simulink model "entire_leg_assembly"  (R2023b)
settings: Solver=ode15s  StartTime=0.0  StopTime=3*(2*length(Wp_1_forward_U)/10)  FixedStep=0.1  MaxStep=1e-3  RelTol=1e-2  AbsTol=1e-5  EnableMultiTasking=on
values from neighbouring files (symbols this model uses):
  Theta1_initial_value = wp_swing(1,1)    [Input_joint_angles.m]
  Theta2_initial_value = wp_swing(2,1)    [Input_joint_angles.m]
  Wp_1_forward_L_3 = repmat(Wp_1_forward_L, 1, 10)    [Input_joint_angles.m]
  Wp_1_forward_U_3 = repmat(Wp_1_forward_U, 1, 10)    [Input_joint_angles.m]
  Wp_3_backward_L_3 = repmat(Wp_3_forward_L, 1, 10)    [Input_joint_angles.m]
  Wp_3_backward_U_3 = repmat(Wp_3_forward_U, 1, 10)    [Input_joint_angles.m]
  Wp_3_forward_L_3 = [1.04719759763 1.04719759763 1.04719759763 1.04719759763 1.04719759763 1.04719759763 1.31601388737 1.31601388737 1.04719759763 1.04719759763 1.04719759763 1.31601388737 ... (1800 elements, 6x300)]    [ForwardWalk.mat]
  Wp_3_forward_U_3 = [-0.523598776024 -0.523598776024 -0.523598776024 -0.523598776024 -0.523598776024 -0.523598776024 -0.649667510569 -0.649667510569 -0.523598776024 -0.523598776024 -0.523598776024 -0.649667510569 ... (1800 elements, 6x300)]    [ForwardWalk.mat]
undefined symbols (not defined in the file or in its folder): X, Y, Z
libraries: sm_lib x76, nesl_utility x25
(part 3 of 3)

== system entire_leg_assembly/Leg3/Leg_LR/Lower_limb1 ==
  Lower_limb : sm_lib/Body Elements/File Solid  Commented=on  ExtGeomFileName=C:\summer 23 thesis om\Robot assembly with 2 linear actuators\Simscape_demo\Leg_lower.STL  UnitType=Custom  ExtGeomFileUnits=mm  StepReaderType=HEX  ExportConvexHullGeometry=off  InertiaType=CalculateFromGeometry  Mass=1.6  MassUnits=kg  CenterOfMass=[0 0 0]  CenterOfMassUnits=m  MomentsOfInertia=[1 1 1]  MomentsOfInertiaUnits=kg*m^2  ProductsOfInertia=[0 0 0]  ProductsOfInertiaUnits=kg*m^2  BasedOnType=Mass  Density=1000  DensityUnits=kg/m^3  DoExposeReferenceFrame=on  SerializedFrames=<Frames><Frame><Id>Frame1</Id><Value><Name>F1</Name><Origin><Source>CenterOfMassFrame</Source><FeatureName></FeatureName></Origin><PrimaryAxis><DefinedDirection>-Y</DefinedDirection><Source>ReferenceFrame</Source><SourceDirection>+Z</SourceDirection><FeatureName></FeatureName></PrimaryAxis><SecondaryAxis><DefinedDirection>+X</DefinedDirection><Source>ReferenceFrame</Source><SourceDirection>+X</SourceDirection><FeatureName></FeatureName></SecondaryAxis></Value></Frame></Frames>  GraphicType=FromGeometry  MarkerShape=Sphere  MarkerSize=10  GraphicVisPropType=SimpleVisualProperties  GraphicDiffuseColor=[0.5 0.5 0.5]  GraphicSpecularColor=[0.5 0.5 0.5 1.0]  GraphicAmbientColor=[0.15 0.15 0.15 1.0]  GraphicEmissiveColor=[0.0 0.0 0.0 1.0]  GraphicShininess=75  GraphicOpacity=1.0
  Lower_limb_OLD : sm_lib/Body Elements/Cylindrical Solid  GraphicAmbientColor=[0.15 0.15 0.15 1.0]  BasedOnType=Density  CenterOfMass=[0 0 0]  CenterOfMassUnits=m  GraphicDiffuseColor=[0.5 0.5 0.5]  CylinderLength=6  CylinderLengthUnits=ft  CylinderRadius=17.46  CylinderRadiusUnits=mm  Density=3000  DensityUnits=kg/m^3  DoExposeReferenceFrame=on  GraphicEmissiveColor=[0.0 0.0 0.0 1.0]  ExportEntireGeometry=on  SerializedFrames=<Frames><Frame><Id>Frame1</Id><Value><Name>F1</Name><Origin><Source>ReferenceFrame</Source><FeatureName></FeatureName></Origin><PrimaryAxis><DefinedDirection>+Y</DefinedDirection><Source>ReferenceFrame</Source><SourceDirection>+Z</SourceDirection><FeatureName></FeatureName></PrimaryAxis><SecondaryAxis><DefinedDirection>+X</DefinedDirection><Source>ReferenceFrame</Source><SourceDirection>+X</SourceDirection><FeatureName></FeatureName></SecondaryAxis></Value></Frame></Frames>  MarkerShape=Sphere  MarkerSize=10  GraphicType=FromGeometry  InertiaType=CalculateFromGeometry  Mass=1  MassUnits=kg  MomentsOfInertia=[1 1 1]  MomentsOfInertiaUnits=kg*m^2  GraphicOpacity=1.0  ProductsOfInertia=[0 0 0]  ProductsOfInertiaUnits=kg*m^2  GraphicShininess=75  GraphicSpecularColor=[0.5 0.5 0.5 1.0]  GraphicVisPropType=SimpleVisualProperties
  Rigid Transform2 : sm_lib/Frames and Transforms/Rigid Transform  TranslationMethod=Cartesian  TranslationStandardOffset=0  TranslationStandardOffsetUnits=m  TranslationStandardAxis=+Z  TranslationCartesianOffset=[0 -3 0]  TranslationCartesianOffsetUnits=ft  TranslationROffset=0  TranslationROffsetUnits=m  TranslationZOffset=0  TranslationZOffsetUnits=m  TranslationThetaOffset=0  TranslationThetaOffsetUnits=deg  RotationMethod=None  RotationAngleUnits=deg  RotationStandardAxis=+Y  RotationAngle=0  RotationArbitraryAxis=[0 0 1]  FollAlignAxisA=+X  BaseAlignAxisA=+Y  FollAlignAxisB=+Y  BaseAlignAxisB=+Z  RotationSequenceAxes=FollowerAxes  RotationSequence=XYX  RotationSequenceAngles=[0 0 0]  RotationSequenceAnglesUnits=deg  RotationMatrix=[1 0 0; 0 1 0; 0 0 1]  Quaternion=[1 0 0 0]
  Conn1 : PMIOPort  Side=Left
  Conn2 : PMIOPort  Port=2  Side=Left
  connections:
  Conn1/RConn1 -- Rigid Transform2/LConn1
  Rigid Transform2/RConn1 -- Lower_limb_OLD/LConn1
  Conn2/RConn1 -- Lower_limb_OLD/LConn2

== system entire_leg_assembly/Leg3/Leg_LR/Upper_limb1 ==
  Rigid Transform : sm_lib/Frames and Transforms/Rigid Transform  TranslationMethod=Cartesian  TranslationStandardOffset=0  TranslationStandardOffsetUnits=m  TranslationStandardAxis=+Z  TranslationCartesianOffset=[0 -3 0]  TranslationCartesianOffsetUnits=ft  TranslationROffset=0  TranslationROffsetUnits=m  TranslationZOffset=0  TranslationZOffsetUnits=m  TranslationThetaOffset=0  TranslationThetaOffsetUnits=deg  RotationMethod=None  RotationAngleUnits=deg  RotationStandardAxis=+Y  RotationAngle=90  RotationArbitraryAxis=[0 0 1]  FollAlignAxisA=+X  BaseAlignAxisA=+Y  FollAlignAxisB=+Y  BaseAlignAxisB=+Z  RotationSequenceAxes=FollowerAxes  RotationSequence=XYX  RotationSequenceAngles=[0 0 0]  RotationSequenceAnglesUnits=deg  RotationMatrix=[1 0 0; 0 1 0; 0 0 1]  Quaternion=[1 0 0 0]
  Rigid Transform1 : sm_lib/Frames and Transforms/Rigid Transform  TranslationMethod=Cartesian  TranslationStandardOffset=0  TranslationStandardOffsetUnits=m  TranslationStandardAxis=+Z  TranslationCartesianOffset=[0 -3 0]  TranslationCartesianOffsetUnits=ft  TranslationROffset=0  TranslationROffsetUnits=m  TranslationZOffset=0  TranslationZOffsetUnits=m  TranslationThetaOffset=0  TranslationThetaOffsetUnits=deg  RotationMethod=None  RotationAngleUnits=deg  RotationStandardAxis=+Z  RotationAngle=0.0  RotationArbitraryAxis=[0 0 1]  FollAlignAxisA=+X  BaseAlignAxisA=+Y  FollAlignAxisB=+Y  BaseAlignAxisB=+Z  RotationSequenceAxes=FollowerAxes  RotationSequence=XYX  RotationSequenceAngles=[0 0 0]  RotationSequenceAnglesUnits=deg  RotationMatrix=[1 0 0; 0 1 0; 0 0 1]  Quaternion=[1 0 0 0]
  Upper_limb : sm_lib/Body Elements/File Solid  ExtGeomFileName=C:\summer 23 thesis om\Robot assembly with 2 linear actuators\Simscape_demo\Leg_upper.STL  UnitType=Custom  ExtGeomFileUnits=mm  StepReaderType=HEX  ExportConvexHullGeometry=off  InertiaType=CalculateFromGeometry  Mass=1.6  MassUnits=kg  CenterOfMass=[0 0 0]  CenterOfMassUnits=m  MomentsOfInertia=[1 1 1]  MomentsOfInertiaUnits=kg*m^2  ProductsOfInertia=[0 0 0]  ProductsOfInertiaUnits=kg*m^2  BasedOnType=Mass  Density=1000  DensityUnits=kg/m^3  DoExposeReferenceFrame=on  SerializedFrames=<Frames><Frame><Id>Frame1</Id><Value><Name>F1</Name><Origin><Source>CenterOfMassFrame</Source><FeatureName></FeatureName></Origin><PrimaryAxis><DefinedDirection>-Y</DefinedDirection><Source>ReferenceFrame</Source><SourceDirection>+Z</SourceDirection><FeatureName></FeatureName></PrimaryAxis><SecondaryAxis><DefinedDirection>+X</DefinedDirection><Source>ReferenceFrame</Source><SourceDirection>+X</SourceDirection><FeatureName></FeatureName></SecondaryAxis></Value></Frame></Frames>  GraphicType=FromGeometry  MarkerShape=Sphere  MarkerSize=10  GraphicVisPropType=SimpleVisualProperties  GraphicDiffuseColor=[0.5 0.5 0.5]  GraphicSpecularColor=[0.5 0.5 0.5 1.0]  GraphicAmbientColor=[0.15 0.15 0.15 1.0]  GraphicEmissiveColor=[0.0 0.0 0.0 1.0]  GraphicShininess=75  GraphicOpacity=1.0
  Conn1 : PMIOPort  Side=Left
  Conn2 : PMIOPort  Port=2  Side=Right
  connections:
  Rigid Transform/LConn1 -- Conn1/RConn1
  Conn2/RConn1 -- Rigid Transform1/RConn1
  Rigid Transform1/LConn1 -- Upper_limb/LConn1 -- Rigid Transform/RConn1

== system entire_leg_assembly/Leg4/Leg_RF/Lower_limb1 ==
  Lower_limb : sm_lib/Body Elements/File Solid  Commented=on  ExtGeomFileName=C:\summer 23 thesis om\Robot assembly with 2 linear actuators\Simscape_demo\Leg_lower.STL  UnitType=Custom  ExtGeomFileUnits=mm  StepReaderType=HEX  ExportConvexHullGeometry=off  InertiaType=CalculateFromGeometry  Mass=1.6  MassUnits=kg  CenterOfMass=[0 0 0]  CenterOfMassUnits=m  MomentsOfInertia=[1 1 1]  MomentsOfInertiaUnits=kg*m^2  ProductsOfInertia=[0 0 0]  ProductsOfInertiaUnits=kg*m^2  BasedOnType=Mass  Density=1000  DensityUnits=kg/m^3  DoExposeReferenceFrame=on  SerializedFrames=<Frames><Frame><Id>Frame1</Id><Value><Name>F1</Name><Origin><Source>CenterOfMassFrame</Source><FeatureName></FeatureName></Origin><PrimaryAxis><DefinedDirection>-Y</DefinedDirection><Source>ReferenceFrame</Source><SourceDirection>+Z</SourceDirection><FeatureName></FeatureName></PrimaryAxis><SecondaryAxis><DefinedDirection>+X</DefinedDirection><Source>ReferenceFrame</Source><SourceDirection>+X</SourceDirection><FeatureName></FeatureName></SecondaryAxis></Value></Frame></Frames>  GraphicType=FromGeometry  MarkerShape=Sphere  MarkerSize=10  GraphicVisPropType=SimpleVisualProperties  GraphicDiffuseColor=[0.5 0.5 0.5]  GraphicSpecularColor=[0.5 0.5 0.5 1.0]  GraphicAmbientColor=[0.15 0.15 0.15 1.0]  GraphicEmissiveColor=[0.0 0.0 0.0 1.0]  GraphicShininess=75  GraphicOpacity=1.0
  Lower_limb_OLD : sm_lib/Body Elements/Cylindrical Solid  GraphicAmbientColor=[0.15 0.15 0.15 1.0]  BasedOnType=Density  CenterOfMass=[0 0 0]  CenterOfMassUnits=m  GraphicDiffuseColor=[0.5 0.5 0.5]  CylinderLength=6  CylinderLengthUnits=ft  CylinderRadius=17.46  CylinderRadiusUnits=mm  Density=3000  DensityUnits=kg/m^3  DoExposeReferenceFrame=on  GraphicEmissiveColor=[0.0 0.0 0.0 1.0]  ExportEntireGeometry=on  SerializedFrames=<Frames><Frame><Id>Frame1</Id><Value><Name>F1</Name><Origin><Source>ReferenceFrame</Source><FeatureName></FeatureName></Origin><PrimaryAxis><DefinedDirection>+Y</DefinedDirection><Source>ReferenceFrame</Source><SourceDirection>+Z</SourceDirection><FeatureName></FeatureName></PrimaryAxis><SecondaryAxis><DefinedDirection>+X</DefinedDirection><Source>ReferenceFrame</Source><SourceDirection>+X</SourceDirection><FeatureName></FeatureName></SecondaryAxis></Value></Frame></Frames>  MarkerShape=Sphere  MarkerSize=10  GraphicType=FromGeometry  InertiaType=CalculateFromGeometry  Mass=1  MassUnits=kg  MomentsOfInertia=[1 1 1]  MomentsOfInertiaUnits=kg*m^2  GraphicOpacity=1.0  ProductsOfInertia=[0 0 0]  ProductsOfInertiaUnits=kg*m^2  GraphicShininess=75  GraphicSpecularColor=[0.5 0.5 0.5 1.0]  GraphicVisPropType=SimpleVisualProperties
  Rigid Transform2 : sm_lib/Frames and Transforms/Rigid Transform  TranslationMethod=Cartesian  TranslationStandardOffset=0  TranslationStandardOffsetUnits=m  TranslationStandardAxis=+Z  TranslationCartesianOffset=[0 -3 0]  TranslationCartesianOffsetUnits=ft  TranslationROffset=0  TranslationROffsetUnits=m  TranslationZOffset=0  TranslationZOffsetUnits=m  TranslationThetaOffset=0  TranslationThetaOffsetUnits=deg  RotationMethod=None  RotationAngleUnits=deg  RotationStandardAxis=+Y  RotationAngle=0  RotationArbitraryAxis=[0 0 1]  FollAlignAxisA=+X  BaseAlignAxisA=+Y  FollAlignAxisB=+Y  BaseAlignAxisB=+Z  RotationSequenceAxes=FollowerAxes  RotationSequence=XYX  RotationSequenceAngles=[0 0 0]  RotationSequenceAnglesUnits=deg  RotationMatrix=[1 0 0; 0 1 0; 0 0 1]  Quaternion=[1 0 0 0]
  Conn1 : PMIOPort  Side=Left
  Connection Port : PMIOPort  Port=2  Side=Left
  connections:
  Conn1/RConn1 -- Rigid Transform2/LConn1
  Rigid Transform2/RConn1 -- Lower_limb_OLD/LConn1
  Lower_limb_OLD/LConn2 -- Connection Port/RConn1

== system entire_leg_assembly/Leg4/Leg_RF/Upper_limb1 ==
  Rigid Transform : sm_lib/Frames and Transforms/Rigid Transform  TranslationMethod=Cartesian  TranslationStandardOffset=0  TranslationStandardOffsetUnits=m  TranslationStandardAxis=+Z  TranslationCartesianOffset=[0 -3 0]  TranslationCartesianOffsetUnits=ft  TranslationROffset=0  TranslationROffsetUnits=m  TranslationZOffset=0  TranslationZOffsetUnits=m  TranslationThetaOffset=0  TranslationThetaOffsetUnits=deg  RotationMethod=None  RotationAngleUnits=deg  RotationStandardAxis=+Y  RotationAngle=90  RotationArbitraryAxis=[0 0 1]  FollAlignAxisA=+X  BaseAlignAxisA=+Y  FollAlignAxisB=+Y  BaseAlignAxisB=+Z  RotationSequenceAxes=FollowerAxes  RotationSequence=XYX  RotationSequenceAngles=[0 0 0]  RotationSequenceAnglesUnits=deg  RotationMatrix=[1 0 0; 0 1 0; 0 0 1]  Quaternion=[1 0 0 0]
  Rigid Transform1 : sm_lib/Frames and Transforms/Rigid Transform  TranslationMethod=Cartesian  TranslationStandardOffset=0  TranslationStandardOffsetUnits=m  TranslationStandardAxis=+Z  TranslationCartesianOffset=[0 -3 0]  TranslationCartesianOffsetUnits=ft  TranslationROffset=0  TranslationROffsetUnits=m  TranslationZOffset=0  TranslationZOffsetUnits=m  TranslationThetaOffset=0  TranslationThetaOffsetUnits=deg  RotationMethod=None  RotationAngleUnits=deg  RotationStandardAxis=+Z  RotationAngle=0.0  RotationArbitraryAxis=[0 0 1]  FollAlignAxisA=+X  BaseAlignAxisA=+Y  FollAlignAxisB=+Y  BaseAlignAxisB=+Z  RotationSequenceAxes=FollowerAxes  RotationSequence=XYX  RotationSequenceAngles=[0 0 0]  RotationSequenceAnglesUnits=deg  RotationMatrix=[1 0 0; 0 1 0; 0 0 1]  Quaternion=[1 0 0 0]
  Upper_limb : sm_lib/Body Elements/File Solid  ExtGeomFileName=C:\summer 23 thesis om\Robot assembly with 2 linear actuators\Simscape_demo\Leg_upper.STL  UnitType=Custom  ExtGeomFileUnits=mm  StepReaderType=HEX  ExportConvexHullGeometry=off  InertiaType=CalculateFromGeometry  Mass=1.6  MassUnits=kg  CenterOfMass=[0 0 0]  CenterOfMassUnits=m  MomentsOfInertia=[1 1 1]  MomentsOfInertiaUnits=kg*m^2  ProductsOfInertia=[0 0 0]  ProductsOfInertiaUnits=kg*m^2  BasedOnType=Mass  Density=1000  DensityUnits=kg/m^3  DoExposeReferenceFrame=on  SerializedFrames=<Frames><Frame><Id>Frame1</Id><Value><Name>F1</Name><Origin><Source>CenterOfMassFrame</Source><FeatureName></FeatureName></Origin><PrimaryAxis><DefinedDirection>-Y</DefinedDirection><Source>ReferenceFrame</Source><SourceDirection>+Z</SourceDirection><FeatureName></FeatureName></PrimaryAxis><SecondaryAxis><DefinedDirection>+X</DefinedDirection><Source>ReferenceFrame</Source><SourceDirection>+X</SourceDirection><FeatureName></FeatureName></SecondaryAxis></Value></Frame></Frames>  GraphicType=FromGeometry  MarkerShape=Sphere  MarkerSize=10  GraphicVisPropType=SimpleVisualProperties  GraphicDiffuseColor=[0.5 0.5 0.5]  GraphicSpecularColor=[0.5 0.5 0.5 1.0]  GraphicAmbientColor=[0.15 0.15 0.15 1.0]  GraphicEmissiveColor=[0.0 0.0 0.0 1.0]  GraphicShininess=75  GraphicOpacity=1.0
  Conn1 : PMIOPort  Side=Left
  Conn2 : PMIOPort  Port=2  Side=Right
  connections:
  Rigid Transform/LConn1 -- Conn1/RConn1
  Conn2/RConn1 -- Rigid Transform1/RConn1
  Rigid Transform1/LConn1 -- Upper_limb/LConn1 -- Rigid Transform/RConn1

== system entire_leg_assembly/Leg5/Leg_RM/Lower_limb1 ==
  Lower_limb : sm_lib/Body Elements/File Solid  Commented=on  ExtGeomFileName=C:\summer 23 thesis om\Robot assembly with 2 linear actuators\Simscape_demo\Leg_lower.STL  UnitType=Custom  ExtGeomFileUnits=mm  StepReaderType=HEX  ExportConvexHullGeometry=off  InertiaType=CalculateFromGeometry  Mass=1.6  MassUnits=kg  CenterOfMass=[0 0 0]  CenterOfMassUnits=m  MomentsOfInertia=[1 1 1]  MomentsOfInertiaUnits=kg*m^2  ProductsOfInertia=[0 0 0]  ProductsOfInertiaUnits=kg*m^2  BasedOnType=Mass  Density=1000  DensityUnits=kg/m^3  DoExposeReferenceFrame=on  SerializedFrames=<Frames><Frame><Id>Frame1</Id><Value><Name>F1</Name><Origin><Source>CenterOfMassFrame</Source><FeatureName></FeatureName></Origin><PrimaryAxis><DefinedDirection>-Y</DefinedDirection><Source>ReferenceFrame</Source><SourceDirection>+Z</SourceDirection><FeatureName></FeatureName></PrimaryAxis><SecondaryAxis><DefinedDirection>+X</DefinedDirection><Source>ReferenceFrame</Source><SourceDirection>+X</SourceDirection><FeatureName></FeatureName></SecondaryAxis></Value></Frame></Frames>  GraphicType=FromGeometry  MarkerShape=Sphere  MarkerSize=10  GraphicVisPropType=SimpleVisualProperties  GraphicDiffuseColor=[0.5 0.5 0.5]  GraphicSpecularColor=[0.5 0.5 0.5 1.0]  GraphicAmbientColor=[0.15 0.15 0.15 1.0]  GraphicEmissiveColor=[0.0 0.0 0.0 1.0]  GraphicShininess=75  GraphicOpacity=1.0
  Lower_limb_OLD : sm_lib/Body Elements/Cylindrical Solid  GraphicAmbientColor=[0.15 0.15 0.15 1.0]  BasedOnType=Density  CenterOfMass=[0 0 0]  CenterOfMassUnits=m  GraphicDiffuseColor=[0.5 0.5 0.5]  CylinderLength=6  CylinderLengthUnits=ft  CylinderRadius=17.46  CylinderRadiusUnits=mm  Density=3000  DensityUnits=kg/m^3  DoExposeReferenceFrame=on  GraphicEmissiveColor=[0.0 0.0 0.0 1.0]  ExportEntireGeometry=on  SerializedFrames=<Frames><Frame><Id>Frame1</Id><Value><Name>F1</Name><Origin><Source>ReferenceFrame</Source><FeatureName></FeatureName></Origin><PrimaryAxis><DefinedDirection>+Y</DefinedDirection><Source>ReferenceFrame</Source><SourceDirection>+Z</SourceDirection><FeatureName></FeatureName></PrimaryAxis><SecondaryAxis><DefinedDirection>+X</DefinedDirection><Source>ReferenceFrame</Source><SourceDirection>+X</SourceDirection><FeatureName></FeatureName></SecondaryAxis></Value></Frame></Frames>  MarkerShape=Sphere  MarkerSize=10  GraphicType=FromGeometry  InertiaType=CalculateFromGeometry  Mass=1  MassUnits=kg  MomentsOfInertia=[1 1 1]  MomentsOfInertiaUnits=kg*m^2  GraphicOpacity=1.0  ProductsOfInertia=[0 0 0]  ProductsOfInertiaUnits=kg*m^2  GraphicShininess=75  GraphicSpecularColor=[0.5 0.5 0.5 1.0]  GraphicVisPropType=SimpleVisualProperties
  Rigid Transform2 : sm_lib/Frames and Transforms/Rigid Transform  TranslationMethod=Cartesian  TranslationStandardOffset=0  TranslationStandardOffsetUnits=m  TranslationStandardAxis=+Z  TranslationCartesianOffset=[0 -3 0]  TranslationCartesianOffsetUnits=ft  TranslationROffset=0  TranslationROffsetUnits=m  TranslationZOffset=0  TranslationZOffsetUnits=m  TranslationThetaOffset=0  TranslationThetaOffsetUnits=deg  RotationMethod=None  RotationAngleUnits=deg  RotationStandardAxis=+Y  RotationAngle=0  RotationArbitraryAxis=[0 0 1]  FollAlignAxisA=+X  BaseAlignAxisA=+Y  FollAlignAxisB=+Y  BaseAlignAxisB=+Z  RotationSequenceAxes=FollowerAxes  RotationSequence=XYX  RotationSequenceAngles=[0 0 0]  RotationSequenceAnglesUnits=deg  RotationMatrix=[1 0 0; 0 1 0; 0 0 1]  Quaternion=[1 0 0 0]
  Conn1 : PMIOPort  Side=Left
  Connection Port : PMIOPort  Port=2  Side=Left
  connections:
  Conn1/RConn1 -- Rigid Transform2/LConn1
  Rigid Transform2/RConn1 -- Lower_limb_OLD/LConn1
  Lower_limb_OLD/LConn2 -- Connection Port/RConn1

== system entire_leg_assembly/Leg5/Leg_RM/Upper_limb1 ==
  Rigid Transform : sm_lib/Frames and Transforms/Rigid Transform  TranslationMethod=Cartesian  TranslationStandardOffset=0  TranslationStandardOffsetUnits=m  TranslationStandardAxis=+Z  TranslationCartesianOffset=[0 -3 0]  TranslationCartesianOffsetUnits=ft  TranslationROffset=0  TranslationROffsetUnits=m  TranslationZOffset=0  TranslationZOffsetUnits=m  TranslationThetaOffset=0  TranslationThetaOffsetUnits=deg  RotationMethod=None  RotationAngleUnits=deg  RotationStandardAxis=+Y  RotationAngle=90  RotationArbitraryAxis=[0 0 1]  FollAlignAxisA=+X  BaseAlignAxisA=+Y  FollAlignAxisB=+Y  BaseAlignAxisB=+Z  RotationSequenceAxes=FollowerAxes  RotationSequence=XYX  RotationSequenceAngles=[0 0 0]  RotationSequenceAnglesUnits=deg  RotationMatrix=[1 0 0; 0 1 0; 0 0 1]  Quaternion=[1 0 0 0]
  Rigid Transform1 : sm_lib/Frames and Transforms/Rigid Transform  TranslationMethod=Cartesian  TranslationStandardOffset=0  TranslationStandardOffsetUnits=m  TranslationStandardAxis=+Z  TranslationCartesianOffset=[0 -3 0]  TranslationCartesianOffsetUnits=ft  TranslationROffset=0  TranslationROffsetUnits=m  TranslationZOffset=0  TranslationZOffsetUnits=m  TranslationThetaOffset=0  TranslationThetaOffsetUnits=deg  RotationMethod=None  RotationAngleUnits=deg  RotationStandardAxis=+Z  RotationAngle=0.0  RotationArbitraryAxis=[0 0 1]  FollAlignAxisA=+X  BaseAlignAxisA=+Y  FollAlignAxisB=+Y  BaseAlignAxisB=+Z  RotationSequenceAxes=FollowerAxes  RotationSequence=XYX  RotationSequenceAngles=[0 0 0]  RotationSequenceAnglesUnits=deg  RotationMatrix=[1 0 0; 0 1 0; 0 0 1]  Quaternion=[1 0 0 0]
  Upper_limb : sm_lib/Body Elements/File Solid  ExtGeomFileName=C:\summer 23 thesis om\Robot assembly with 2 linear actuators\Simscape_demo\Leg_upper.STL  UnitType=Custom  ExtGeomFileUnits=mm  StepReaderType=HEX  ExportConvexHullGeometry=off  InertiaType=CalculateFromGeometry  Mass=1.6  MassUnits=kg  CenterOfMass=[0 0 0]  CenterOfMassUnits=m  MomentsOfInertia=[1 1 1]  MomentsOfInertiaUnits=kg*m^2  ProductsOfInertia=[0 0 0]  ProductsOfInertiaUnits=kg*m^2  BasedOnType=Mass  Density=1000  DensityUnits=kg/m^3  DoExposeReferenceFrame=on  SerializedFrames=<Frames><Frame><Id>Frame1</Id><Value><Name>F1</Name><Origin><Source>CenterOfMassFrame</Source><FeatureName></FeatureName></Origin><PrimaryAxis><DefinedDirection>-Y</DefinedDirection><Source>ReferenceFrame</Source><SourceDirection>+Z</SourceDirection><FeatureName></FeatureName></PrimaryAxis><SecondaryAxis><DefinedDirection>+X</DefinedDirection><Source>ReferenceFrame</Source><SourceDirection>+X</SourceDirection><FeatureName></FeatureName></SecondaryAxis></Value></Frame></Frames>  GraphicType=FromGeometry  MarkerShape=Sphere  MarkerSize=10  GraphicVisPropType=SimpleVisualProperties  GraphicDiffuseColor=[0.5 0.5 0.5]  GraphicSpecularColor=[0.5 0.5 0.5 1.0]  GraphicAmbientColor=[0.15 0.15 0.15 1.0]  GraphicEmissiveColor=[0.0 0.0 0.0 1.0]  GraphicShininess=75  GraphicOpacity=1.0
  Conn1 : PMIOPort  Side=Left
  Conn2 : PMIOPort  Port=2  Side=Right
  connections:
  Rigid Transform/LConn1 -- Conn1/RConn1
  Conn2/RConn1 -- Rigid Transform1/RConn1
  Rigid Transform1/LConn1 -- Upper_limb/LConn1 -- Rigid Transform/RConn1

== system entire_leg_assembly/Leg6/Leg_RB/Lower_limb1 ==
  Lower_limb : sm_lib/Body Elements/File Solid  Commented=on  ExtGeomFileName=C:\summer 23 thesis om\Robot assembly with 2 linear actuators\Simscape_demo\Leg_lower.STL  UnitType=Custom  ExtGeomFileUnits=mm  StepReaderType=HEX  ExportConvexHullGeometry=off  InertiaType=CalculateFromGeometry  Mass=1.6  MassUnits=kg  CenterOfMass=[0 0 0]  CenterOfMassUnits=m  MomentsOfInertia=[1 1 1]  MomentsOfInertiaUnits=kg*m^2  ProductsOfInertia=[0 0 0]  ProductsOfInertiaUnits=kg*m^2  BasedOnType=Mass  Density=1000  DensityUnits=kg/m^3  DoExposeReferenceFrame=on  SerializedFrames=<Frames><Frame><Id>Frame1</Id><Value><Name>F1</Name><Origin><Source>CenterOfMassFrame</Source><FeatureName></FeatureName></Origin><PrimaryAxis><DefinedDirection>-Y</DefinedDirection><Source>ReferenceFrame</Source><SourceDirection>+Z</SourceDirection><FeatureName></FeatureName></PrimaryAxis><SecondaryAxis><DefinedDirection>+X</DefinedDirection><Source>ReferenceFrame</Source><SourceDirection>+X</SourceDirection><FeatureName></FeatureName></SecondaryAxis></Value></Frame></Frames>  GraphicType=FromGeometry  MarkerShape=Sphere  MarkerSize=10  GraphicVisPropType=SimpleVisualProperties  GraphicDiffuseColor=[0.5 0.5 0.5]  GraphicSpecularColor=[0.5 0.5 0.5 1.0]  GraphicAmbientColor=[0.15 0.15 0.15 1.0]  GraphicEmissiveColor=[0.0 0.0 0.0 1.0]  GraphicShininess=75  GraphicOpacity=1.0
  Lower_limb_OLD : sm_lib/Body Elements/Cylindrical Solid  GraphicAmbientColor=[0.15 0.15 0.15 1.0]  BasedOnType=Density  CenterOfMass=[0 0 0]  CenterOfMassUnits=m  GraphicDiffuseColor=[0.5 0.5 0.5]  CylinderLength=6  CylinderLengthUnits=ft  CylinderRadius=17.46  CylinderRadiusUnits=mm  Density=3000  DensityUnits=kg/m^3  DoExposeReferenceFrame=on  GraphicEmissiveColor=[0.0 0.0 0.0 1.0]  ExportEntireGeometry=on  SerializedFrames=<Frames><Frame><Id>Frame1</Id><Value><Name>F1</Name><Origin><Source>ReferenceFrame</Source><FeatureName></FeatureName></Origin><PrimaryAxis><DefinedDirection>+Y</DefinedDirection><Source>ReferenceFrame</Source><SourceDirection>+Z</SourceDirection><FeatureName></FeatureName></PrimaryAxis><SecondaryAxis><DefinedDirection>+X</DefinedDirection><Source>ReferenceFrame</Source><SourceDirection>+X</SourceDirection><FeatureName></FeatureName></SecondaryAxis></Value></Frame></Frames>  MarkerShape=Sphere  MarkerSize=10  GraphicType=FromGeometry  InertiaType=CalculateFromGeometry  Mass=1  MassUnits=kg  MomentsOfInertia=[1 1 1]  MomentsOfInertiaUnits=kg*m^2  GraphicOpacity=1.0  ProductsOfInertia=[0 0 0]  ProductsOfInertiaUnits=kg*m^2  GraphicShininess=75  GraphicSpecularColor=[0.5 0.5 0.5 1.0]  GraphicVisPropType=SimpleVisualProperties
  Rigid Transform2 : sm_lib/Frames and Transforms/Rigid Transform  TranslationMethod=Cartesian  TranslationStandardOffset=0  TranslationStandardOffsetUnits=m  TranslationStandardAxis=+Z  TranslationCartesianOffset=[0 -3 0]  TranslationCartesianOffsetUnits=ft  TranslationROffset=0  TranslationROffsetUnits=m  TranslationZOffset=0  TranslationZOffsetUnits=m  TranslationThetaOffset=0  TranslationThetaOffsetUnits=deg  RotationMethod=None  RotationAngleUnits=deg  RotationStandardAxis=+Y  RotationAngle=0  RotationArbitraryAxis=[0 0 1]  FollAlignAxisA=+X  BaseAlignAxisA=+Y  FollAlignAxisB=+Y  BaseAlignAxisB=+Z  RotationSequenceAxes=FollowerAxes  RotationSequence=XYX  RotationSequenceAngles=[0 0 0]  RotationSequenceAnglesUnits=deg  RotationMatrix=[1 0 0; 0 1 0; 0 0 1]  Quaternion=[1 0 0 0]
  Conn1 : PMIOPort  Side=Left
  Connection Port : PMIOPort  Port=2  Side=Left
  connections:
  Conn1/RConn1 -- Rigid Transform2/LConn1
  Rigid Transform2/RConn1 -- Lower_limb_OLD/LConn1
  Lower_limb_OLD/LConn2 -- Connection Port/RConn1

== system entire_leg_assembly/Leg6/Leg_RB/Upper_limb1 ==
  Rigid Transform : sm_lib/Frames and Transforms/Rigid Transform  TranslationMethod=Cartesian  TranslationStandardOffset=0  TranslationStandardOffsetUnits=m  TranslationStandardAxis=+Z  TranslationCartesianOffset=[0 -3 0]  TranslationCartesianOffsetUnits=ft  TranslationROffset=0  TranslationROffsetUnits=m  TranslationZOffset=0  TranslationZOffsetUnits=m  TranslationThetaOffset=0  TranslationThetaOffsetUnits=deg  RotationMethod=None  RotationAngleUnits=deg  RotationStandardAxis=+Y  RotationAngle=90  RotationArbitraryAxis=[0 0 1]  FollAlignAxisA=+X  BaseAlignAxisA=+Y  FollAlignAxisB=+Y  BaseAlignAxisB=+Z  RotationSequenceAxes=FollowerAxes  RotationSequence=XYX  RotationSequenceAngles=[0 0 0]  RotationSequenceAnglesUnits=deg  RotationMatrix=[1 0 0; 0 1 0; 0 0 1]  Quaternion=[1 0 0 0]
  Rigid Transform1 : sm_lib/Frames and Transforms/Rigid Transform  TranslationMethod=Cartesian  TranslationStandardOffset=0  TranslationStandardOffsetUnits=m  TranslationStandardAxis=+Z  TranslationCartesianOffset=[0 -3 0]  TranslationCartesianOffsetUnits=ft  TranslationROffset=0  TranslationROffsetUnits=m  TranslationZOffset=0  TranslationZOffsetUnits=m  TranslationThetaOffset=0  TranslationThetaOffsetUnits=deg  RotationMethod=None  RotationAngleUnits=deg  RotationStandardAxis=+Z  RotationAngle=0.0  RotationArbitraryAxis=[0 0 1]  FollAlignAxisA=+X  BaseAlignAxisA=+Y  FollAlignAxisB=+Y  BaseAlignAxisB=+Z  RotationSequenceAxes=FollowerAxes  RotationSequence=XYX  RotationSequenceAngles=[0 0 0]  RotationSequenceAnglesUnits=deg  RotationMatrix=[1 0 0; 0 1 0; 0 0 1]  Quaternion=[1 0 0 0]
  Upper_limb : sm_lib/Body Elements/File Solid  ExtGeomFileName=C:\summer 23 thesis om\Robot assembly with 2 linear actuators\Simscape_demo\Leg_upper.STL  UnitType=Custom  ExtGeomFileUnits=mm  StepReaderType=HEX  ExportConvexHullGeometry=off  InertiaType=CalculateFromGeometry  Mass=1.6  MassUnits=kg  CenterOfMass=[0 0 0]  CenterOfMassUnits=m  MomentsOfInertia=[1 1 1]  MomentsOfInertiaUnits=kg*m^2  ProductsOfInertia=[0 0 0]  ProductsOfInertiaUnits=kg*m^2  BasedOnType=Mass  Density=1000  DensityUnits=kg/m^3  DoExposeReferenceFrame=on  SerializedFrames=<Frames><Frame><Id>Frame1</Id><Value><Name>F1</Name><Origin><Source>CenterOfMassFrame</Source><FeatureName></FeatureName></Origin><PrimaryAxis><DefinedDirection>-Y</DefinedDirection><Source>ReferenceFrame</Source><SourceDirection>+Z</SourceDirection><FeatureName></FeatureName></PrimaryAxis><SecondaryAxis><DefinedDirection>+X</DefinedDirection><Source>ReferenceFrame</Source><SourceDirection>+X</SourceDirection><FeatureName></FeatureName></SecondaryAxis></Value></Frame></Frames>  GraphicType=FromGeometry  MarkerShape=Sphere  MarkerSize=10  GraphicVisPropType=SimpleVisualProperties  GraphicDiffuseColor=[0.5 0.5 0.5]  GraphicSpecularColor=[0.5 0.5 0.5 1.0]  GraphicAmbientColor=[0.15 0.15 0.15 1.0]  GraphicEmissiveColor=[0.0 0.0 0.0 1.0]  GraphicShininess=75  GraphicOpacity=1.0
  Conn1 : PMIOPort  Side=Left
  Conn2 : PMIOPort  Port=2  Side=Right
  connections:
  Rigid Transform/LConn1 -- Conn1/RConn1
  Conn2/RConn1 -- Rigid Transform1/RConn1
  Rigid Transform1/LConn1 -- Upper_limb/LConn1 -- Rigid Transform/RConn1

== matlab function entire_leg_assembly/Signal Generator2/MATLAB Function ==
  settings: updateMethod=DISCRETE
  data: t input; U1_theta1 output; U2_theta1 output; Wp_1_forward_U input; Wp_3_backward_U_3 input; Wp_1_forward_L input; Wp_3_backward_L_3 input; U3_theta1 output; U4_theta1 output; U5_theta1 output; U6_theta1 output; L1_theta1 output; L2_theta1 output; L3_theta1 output; L4_theta1 output; L5_theta1 output; L6_theta1 output; Theta1_initial_value input; Theta2_initial_value input
function [U1_theta1,U2_theta1,U3_theta1,U4_theta1,U5_theta1,U6_theta1,L1_theta1, L2_theta1,L3_theta1,L4_theta1, L5_theta1, L6_theta1] = SignalGenerator(t, Wp_1_forward_U, Wp_3_backward_U_3, Wp_1_forward_L, Wp_3_backward_L_3, Theta1_initial_value, Theta2_initial_value)
%     % Define the time array and joint angles
% %UPPER LIMB ANGLES    
%     persistent U1_t1
%     if isempty(U1_t1)
%        U1_t1 = Theta1_initial_value;
%     end
% 
%     persistent U2_t1
%     if isempty(U2_t1)
%        U2_t1 = Theta1_initial_value;
%     end
% 
%       persistent U3_t1
%     if isempty(U3_t1)
%        U3_t1 = Theta1_initial_value;
%     end
% 
%     persistent U4_t1
%     if isempty(U4_t1)
%        U4_t1 = Theta1_initial_value;
%     end
% 
% 
%   persistent U5_t1
%     if isempty(U5_t1)
%        U5_t1 = Theta1_initial_value;
%     end
% 
%     persistent U6_t1
%     if isempty(U6_t1)
%        U6_t1 = Theta1_initial_value;
%     end
% 
% %LOWER LIMB ANGLES
%     persistent L1_t1
%     if isempty(L1_t1)
%        L1_t1 = Theta1_initial_value;
%     end
% 
%     persistent L2_t1
%     if isempty(L2_t1)
%        L2_t1 = Theta1_initial_value;
%     end
% 
%       persistent L3_t1
%     if isempty(L3_t1)
%        L3_t1 = Theta1_initial_value;
%     end
% 
%     persistent L4_t1
%     if isempty(L4_t1)
%        L4_t1 = Theta1_initial_value;
%     end
% 
% 
%   persistent L5_t1
%     if isempty(L5_t1)
%        L5_t1 = Theta1_initial_value;
%     end
% 
%     persistent L6_t1
%     if isempty(L6_t1)
%        L6_t1 = Theta1_initial_value;
%     end
% 
%    persistent index
%    if isempty(index)
%        index = 1;
%    end
% 
% 
%    index    
% 
%    U1_t1 = Wp_1_forward_U(1,index);
%    U2_t1 = Wp_1_forward_U(2,index);
%    U3_t1 = Wp_1_forward_U(3,index);       
%    U4_t1 = Wp_1_forward_U(4,index);
%    U5_t1 = Wp_1_forward_U(5,index);
%    U6_t1 = Wp_1_forward_U(6,index);
%    L1_t1 = Wp_1_forward_L(1,index);
%    L2_t1 = Wp_1_forward_L(2,index);
%    L3_t1 = Wp_1_forward_L(3,index);
%    L4_t1 = Wp_1_forward_L(4,index);
%    L5_t1 = Wp_1_forward_L(5,index);
%    L6_t1 = Wp_1_forward_L(6,index);
% 
% 
% 
% 
% 
%     % Interpolate the joint angle based on time(Upper leg)
%     U1_theta1 = U1_t1;
%     U2_theta1 = U2_t1;
%     U3_theta1 = U3_t1;
%     U4_theta1 = U4_t1;
%     U5_theta1 = U5_t1;
%     U6_theta1 = U6_t1;
% 
% 
% 
%  % Interpolate the joint angle based on time(Lower leg)
%     L1_theta1 = L1_t1;
%     L2_theta1 = L2_t1;
%     L3_theta1 = L3_t1;
%     L4_theta1 = L4_t1;
%     L5_theta1 = L5_t1;
%     L6_theta1 = L6_t1;
% 
% index = index +1;

   %time_vector = round(linspace(0,2*length(Wp_1_forward_U)/10,length(Wp_1_forward_U)),1);  % 6 steps for 10 seconds
   time_vector = 0 : 0.2 : (0.2 * 299);  % 70 elements total
   %length(time_vector)


    % Interpolate the joint angle based on time(Upper leg)
    U1_theta1 = interp1(time_vector, Wp_1_forward_U(1,(1:end)), t, 'linear', 'extrap'); %Upper leg joint angle leg1
    U2_theta1 = interp1(time_vector, Wp_3_backward_U_3(3,(1:end)), t, 'linear', 'extrap'); %Upper leg joint angle leg2
    U3_theta1 = interp1(time_vector, Wp_1_forward_U(2,(1:end)), t, 'linear', 'extrap'); %Upper leg joint angle leg3
    U4_theta1 = interp1(time_vector,  Wp_3_backward_U_3(4,(1:end)), t, 'linear', 'extrap'); %Upper leg joint angle leg4
    U5_theta1 = interp1(time_vector, Wp_1_forward_U(6,(1:end)), t, 'linear', 'extrap'); %Upper leg joint angle leg5
    U6_theta1 = interp1(time_vector,  Wp_3_backward_U_3(5,(1:end)), t, 'linear', 'extrap'); %Upper leg joint angle leg6



 % Interpolate the joint angle based on time(Lower leg)
    L1_theta1 = interp1(time_vector, Wp_1_forward_L(1,(1:end)), t, 'linear', 'extrap'); %Lower leg joint angle leg1
    L2_theta1 = interp1(time_vector, Wp_3_backward_L_3(3,(1:end)), t, 'linear', 'extrap'); %Lower leg joint angle leg2
    L3_theta1 = interp1(time_vector, Wp_1_forward_L(2,(1:end)), t, 'linear', 'extrap'); %Lower leg joint angle leg3
    L4_theta1 = interp1(time_vector, Wp_3_backward_L_3(4,(1:end)), t, 'linear', 'extrap'); %Lower leg joint angle leg4
    L5_theta1 = interp1(time_vector, Wp_1_forward_L(6,(1:end)), t, 'linear', 'extrap'); %Lower leg joint angle leg5
    L6_theta1 = interp1(time_vector, Wp_3_backward_L_3(5,(1:end)), t, 'linear', 'extrap'); %Lower leg joint angle leg6

== matlab function entire_leg_assembly/Signal Generator/MATLAB Function ==
  settings: updateMethod=DISCRETE
  data: t input; U1_theta1 output; U2_theta1 output; Wp_1_forward_U input; Wp_1_forward_L input; U3_theta1 output; U4_theta1 output; U5_theta1 output; U6_theta1 output; L1_theta1 output; L2_theta1 output; L3_theta1 output; L4_theta1 output; L5_theta1 output; L6_theta1 output; Theta1_initial_value input; Theta2_initial_value input
function [U1_theta1,U2_theta1,U3_theta1,U4_theta1,U5_theta1,U6_theta1,L1_theta1, L2_theta1,L3_theta1,L4_theta1, L5_theta1, L6_theta1] = SignalGenerator(t, Wp_1_forward_U, Wp_1_forward_L, Theta1_initial_value, Theta2_initial_value)
%     % Define the time array and joint angles
% %UPPER LIMB ANGLES    
%     persistent U1_t1
%     if isempty(U1_t1)
%        U1_t1 = Theta1_initial_value;
%     end
% 
%     persistent U2_t1
%     if isempty(U2_t1)
%        U2_t1 = Theta1_initial_value;
%     end
% 
%       persistent U3_t1
%     if isempty(U3_t1)
%        U3_t1 = Theta1_initial_value;
%     end
% 
%     persistent U4_t1
%     if isempty(U4_t1)
%        U4_t1 = Theta1_initial_value;
%     end
% 
% 
%   persistent U5_t1
%     if isempty(U5_t1)
%        U5_t1 = Theta1_initial_value;
%     end
% 
%     persistent U6_t1
%     if isempty(U6_t1)
%        U6_t1 = Theta1_initial_value;
%     end
% 
% %LOWER LIMB ANGLES
%     persistent L1_t1
%     if isempty(L1_t1)
%        L1_t1 = Theta1_initial_value;
%     end
% 
%     persistent L2_t1
%     if isempty(L2_t1)
%        L2_t1 = Theta1_initial_value;
%     end
% 
%       persistent L3_t1
%     if isempty(L3_t1)
%        L3_t1 = Theta1_initial_value;
%     end
% 
%     persistent L4_t1
%     if isempty(L4_t1)
%        L4_t1 = Theta1_initial_value;
%     end
% 
% 
%   persistent L5_t1
%     if isempty(L5_t1)
%        L5_t1 = Theta1_initial_value;
%     end
% 
%     persistent L6_t1
%     if isempty(L6_t1)
%        L6_t1 = Theta1_initial_value;
%     end
% 
%    persistent index
%    if isempty(index)
%        index = 1;
%    end
% 
% 
%    index    
% 
%    U1_t1 = Wp_1_forward_U(1,index);
%    U2_t1 = Wp_1_forward_U(2,index);
%    U3_t1 = Wp_1_forward_U(3,index);       
%    U4_t1 = Wp_1_forward_U(4,index);
%    U5_t1 = Wp_1_forward_U(5,index);
%    U6_t1 = Wp_1_forward_U(6,index);
%    L1_t1 = Wp_1_forward_L(1,index);
%    L2_t1 = Wp_1_forward_L(2,index);
%    L3_t1 = Wp_1_forward_L(3,index);
%    L4_t1 = Wp_1_forward_L(4,index);
%    L5_t1 = Wp_1_forward_L(5,index);
%    L6_t1 = Wp_1_forward_L(6,index);
% 
% 
% 
% 
% 
%     % Interpolate the joint angle based on time(Upper leg)
%     U1_theta1 = U1_t1;
%     U2_theta1 = U2_t1;
%     U3_theta1 = U3_t1;
%     U4_theta1 = U4_t1;
%     U5_theta1 = U5_t1;
%     U6_theta1 = U6_t1;
% 
% 
% 
%  % Interpolate the joint angle based on time(Lower leg)
%     L1_theta1 = L1_t1;
%     L2_theta1 = L2_t1;
%     L3_theta1 = L3_t1;
%     L4_theta1 = L4_t1;
%     L5_theta1 = L5_t1;
%     L6_theta1 = L6_t1;
% 
% index = index +1;

   %time_vector = round(linspace(0,2*length(Wp_1_forward_U)/10,length(Wp_1_forward_U)),1);  % 6 steps for 10 seconds
   time_vector = 0 : 0.2 : (0.2 * 209);  % 70 elements total



    % Interpolate the joint angle based on time(Upper leg)
    U1_theta1 = interp1(time_vector, Wp_1_forward_U(1,(1:end)), t, 'linear', 'extrap'); %Upper leg joint angle leg1
    U2_theta1 = interp1(time_vector, Wp_1_forward_U(2,(1:end)), t, 'linear', 'extrap'); %Upper leg joint angle leg2
    U3_theta1 = interp1(time_vector, Wp_1_forward_U(3,(1:end)), t, 'linear', 'extrap'); %Upper leg joint angle leg3
    U4_theta1 = interp1(time_vector, Wp_1_forward_U(4,(1:end)), t, 'linear', 'extrap'); %Upper leg joint angle leg4
    U5_theta1 = interp1(time_vector, Wp_1_forward_U(5,(1:end)), t, 'linear', 'extrap'); %Upper leg joint angle leg5
    U6_theta1 = interp1(time_vector, Wp_1_forward_U(6,(1:end)), t, 'linear', 'extrap'); %Upper leg joint angle leg6



 % Interpolate the joint angle based on time(Lower leg)
    L1_theta1 = interp1(time_vector, Wp_1_forward_L(1,(1:end)), t, 'linear', 'extrap'); %Lower leg joint angle leg1
    L2_theta1 = interp1(time_vector, Wp_1_forward_L(2,(1:end)), t, 'linear', 'extrap'); %Lower leg joint angle leg2
    L3_theta1 = interp1(time_vector, Wp_1_forward_L(3,(1:end)), t, 'linear', 'extrap'); %Lower leg joint angle leg3
    L4_theta1 = interp1(time_vector, Wp_1_forward_L(4,(1:end)), t, 'linear', 'extrap'); %Lower leg joint angle leg4
    L5_theta1 = interp1(time_vector, Wp_1_forward_L(5,(1:end)), t, 'linear', 'extrap'); %Lower leg joint angle leg5
    L6_theta1 = interp1(time_vector, Wp_1_forward_L(6,(1:end)), t, 'linear', 'extrap'); %Lower leg joint angle leg6
